simulink model "BPM_VA_Agitation_sfun_xk"  (R2022b)
settings: configuration reference "ModelConfig_var" (kept outside this file)
InitFcn:
  | %% BUS initialization
  | Xabc.A = 0;
  | Xabc.B = 0;
  | Xabc.C = 0;
  | % -------------------------------------------------------------------------
  | Simulink.Bus.createObject(Xabc)
  | XabcBus = slBus1;
  | clear slBus1
  | 
  | %% Parameter Structure initialization
  | Motor_prm_init_bpm;
model workspace (MAT data in the model file):
  Mech_HAs_CF = 0
  Mech_HAs_J_drum = 0
  Mech_HAs_TR = 0
  Mech_HAs_damp = 0
  Mech_HAs_m_unb = 0
  Mech_HAs_r_unb = 0
  Mech_VAa_J_basket = 0
  Mech_VAa_J_impeller = 0
  Mech_VAa_basket_dens = 0
  Mech_VAa_basket_dia = 0
  Mech_VAa_belt_ratio = 0
  Mech_VAa_clothes_mass = 0
  Mech_VAa_gear_ratio = 0
  Mech_VAa_imp_dens = 0
  Mech_VAa_water_vol = 0
  Mech_VAs_D_r = 0
  Mech_VAs_I_zt = 0
  Mech_VAs_K = 2700
  Mech_VAs_T_f = 0
  Mech_VAs_belt_rat = 0
  Mech_VAs_d = 0
  Mech_VAs_e = 0
  Mech_VAs_m_b1 = 0
  Mech_VAs_m_b2 = 0
  Mech_VAs_m_d = 0
  Mech_VAs_m_t = 0
  Mech_VAs_m_u = 0
  Time_step = 0.0001
  Time_step_solver = 0
  bpm_B = 0
  bpm_Ipk = [0 1 2 3 4 5 6 7]
  bpm_Jrotor = 0
  bpm_Ld_0 = 0.02117
  bpm_Ld_a = [0.02117 0.02117 0.02117 0.02117 0.02117 0.02117 0.02117 0.02117]
  bpm_Loss_Power = [0 1 2 3 4 5 6 7]
  bpm_Loss_Speed = [0 1 2 3 4 5 6 7]
  bpm_Loss_flag = 1
  bpm_Loss_th = 10
  bpm_Lq_0 = 0.02117
  bpm_Lq_b = [0.02117 0.02117 0.02117 0.02117 0.02117 0.02117 0.02117 0.02117]
  bpm_Ls_sat_flag = 1
  bpm_NPP = 0
  bpm_PM_flux_h1_0 = 0
  bpm_PM_rotor_alpha = 0
  bpm_Rs_0 = 0
  bpm_Rs_stator_alpha = 0
  bpm_Rsa_aux = 0
  bpm_Rsb_aux = 0
  bpm_Rsc_aux = 0
  bpm_TR = 1
  bpm_Temp_rotor_0 = 0
  bpm_Temp_stator_0 = 0
libraries: bpm_dq_S_noH_D_RL_U_VA_Agitation_xk x1
settings Model: ParameterArgumentNames=Mech_HAs_CF,Mech_HAs_J_drum,Mech_HAs_TR,Mech_HAs_damp,Mech_HAs_m_unb,Mech_HAs_r_unb,Mech_VAa_J_basket,Mech_VAa_J_impeller,Mech_VAa_basket_dens,Mech_VAa_basket_dia,Mech_VAa_belt_ratio,Mech_VAa_clothes_mass,Mech_VAa_gear_ratio,Mech_VAa_imp_dens,Mech_VAa_water_vol,Mech_VAs_D_r,Mech_VAs_I_zt,Mech_VAs_K,Mech_VAs_T_f,Mech_VAs_belt_rat,Mech_VAs_d,Mech_VAs_e,Mech_VAs_m_b1,Mech_VAs_m_b2,Mech_VAs_m_d,Mech_VAs_m_t,Mech_VAs_m_u,Time_step_solver,bpm_B,bpm_Ipk,bpm_Jrotor,bpm_Ld_0,bpm_Ld_a,bpm_Loss_Power,bpm_Loss_Speed,bpm_Loss_flag,bpm_Loss_th,bpm_Lq_0,bpm_Lq_b,bpm_Ls_sat_flag,bpm_NPP,bpm_PM_flux_h1_0,bpm_PM_rotor_alpha,bpm_Rs_0,bpm_Rs_stator_alpha,bpm_Rsa_aux,bpm_Rsb_aux,bpm_Rsc_aux,bpm_TR,bpm_Temp_rotor_0,bpm_Temp_stator_0  Creator=BEDNASA  LastModifiedBy=BEDNASA
settings ConfigSetRef: SourceName=ModelConfig_var  SourceLocation=Base Workspace

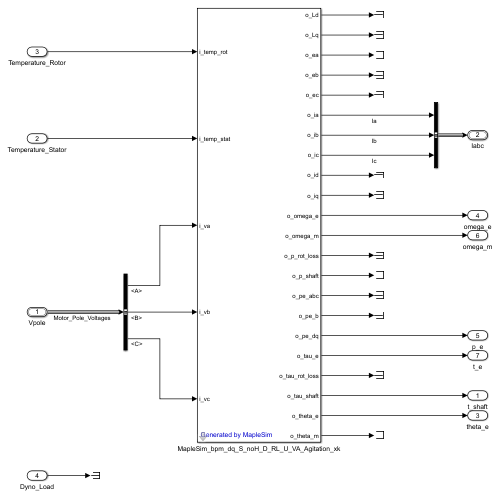
[thumbnail: Simulink's stored preview of the top-level diagram]
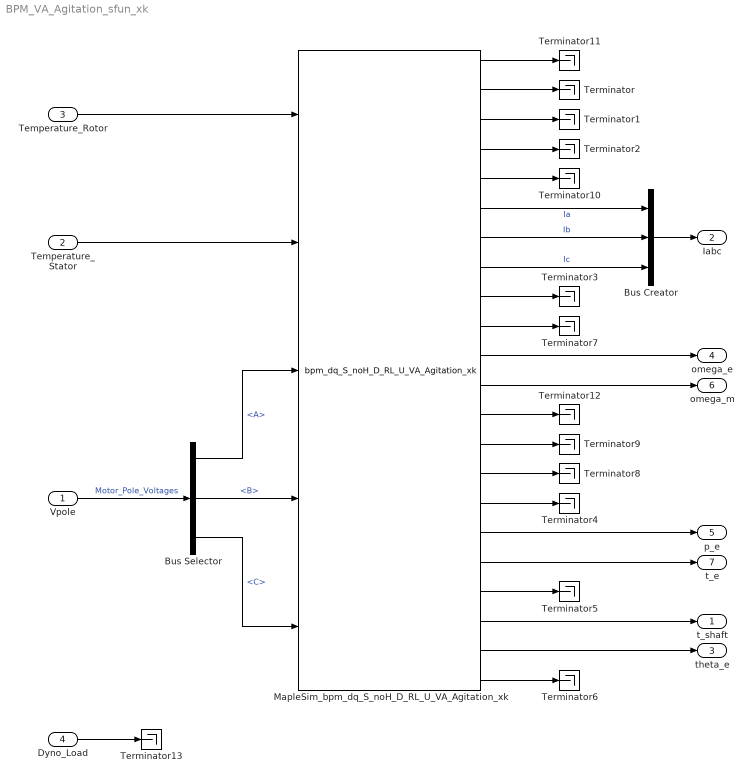
== system BPM_VA_Agitation_sfun_xk ==
  Vpole : Inport  OutDataTypeStr=Bus: XabcBus
  Temperature_Stator : Inport  Port=2
  Temperature_Rotor : Inport  Port=3
  Dyno_Load : Inport  Port=4
  Bus Creator : BusCreator  Inputs=3
  Bus Selector : BusSelector  OutputSignals=A,B,C
  MapleSim_bpm_dq_S_noH_D_RL_U_VA_Agitation_xk : bpm_dq_S_noH_D_RL_U_VA_Agitation_xk/bpm_dq_S_noH_D_RL_U_VA_Agitation_xk  Description=Subsystem: MapleSim_bpm_dq_S_noH_D_RL_U_VA_Agitation_xk  ic=[-0., 0., -0., 0., -0., 0., -0., 0., -0., 0., 0., 0., 0., 0.]  Par1=bpm_B  Par2=bpm_Ipk(1)  Par3=bpm_Ipk(2)  Par4=bpm_Ipk(3)  Par5=bpm_Ipk(4)  Par6=bpm_Ipk(5)  Par7=bpm_Ipk(6)  Par8=bpm_Ipk(7)  Par9=bpm_Ipk(8)  Par10=bpm_Jrotor  Par11=bpm_Ld_0  Par12=bpm_Ld_a(1)  Par13=bpm_Ld_a(2)  Par14=bpm_Ld_a(3)  Par15=bpm_Ld_a(4)  Par16=bpm_Ld_a(5)  Par17=bpm_Ld_a(6)  Par18=bpm_Ld_a(7)  Par19=bpm_Ld_a(8)  Par20=bpm_Lq_0  Par21=bpm_Lq_b(1)  Par22=bpm_Lq_b(2)  Par23=bpm_Lq_b(3)  Par24=bpm_Lq_b(4)  Par25=bpm_Lq_b(5)  Par26=bpm_Lq_b(6)  Par27=bpm_Lq_b(7)  Par28=bpm_Lq_b(8)  Par29=bpm_Ls_sat_flag  Par30=bpm_NPP  Par31=bpm_Loss_Power(1)  Par32=bpm_Loss_Power(2)  Par33=bpm_Loss_Power(3)  Par34=bpm_Loss_Power(4)  Par35=bpm_Loss_Power(5)  Par36=bpm_Loss_Power(6)  Par37=bpm_Loss_Power(7)  Par38=bpm_Loss_Power(8)  Par39=bpm_Loss_Speed(1)  Par40=bpm_Loss_Speed(2)  Par41=bpm_Loss_Speed(3)  Par42=bpm_Loss_Speed(4)  Par43=bpm_Loss_Speed(5)  Par44=bpm_Loss_Speed(6)  Par45=bpm_Loss_Speed(7)  Par46=bpm_Loss_Speed(8)  Par47=bpm_Loss_flag  Par48=bpm_Loss_th  Par49=bpm_Rs_0  Par50=bpm_Rsa_aux  Par51=bpm_Rsb_aux  Par52=bpm_Rsc_aux  Par53=bpm_Temp_rotor_0  Par54=bpm_Temp_stator_0  Par55=Time_step_solver  Par56=bpm_Rs_stator_alpha  Par57=bpm_PM_rotor_alpha  Par58=bpm_PM_flux_h1_0  Par59=Mech_VAa_basket_dia  Par60=Mech_VAa_clothes_mass  Par61=4.23681450081440905  Par62=5.78489261990852491  Par63=.130062059062488242  Par64=2.51144671645133697  Par65=.813472814676472229e-2  Par66=52.1060414955483938  Par67=Mech_VAa_J_basket  Par68=Mech_VAa_J_impeller  Par69=1.4270582175789073  Par70=12.0291903656936093  Par71=6.33381904348042595  Par72=2.3559208849248882  Par73=3.07609149344609313  Par74=3.16664968265920829  Par75=Mech_VAa_belt_ratio  Par76=.501051232161794397  Par77=.500198165205360073  Par78=.519008970935830595  Par79=.502279004521981584  Par80=0.  Par81=Mech_VAa_gear_ratio  Par82=0.  Par83=0.  Par84=0.  Par85=0.  Par86=0.  Par87=0.  Par88=Mech_VAa_water_vol  MinStep=1/40  TimeStep_Solver=TimeSteps.ModelStep
      settings: LibrarySourceBlock=MapleSim_bpm_dq_S_noH_D_RL_U_VA_Agitation_xk/MapleSim_bpm_dq_S_noH_D_RL_U_VA_Agitation_xk
  Terminator{,1..13} (14 alike) : Terminator
  t_shaft : Outport  VectorParamsAs1DForOutWhenUnconnected=off
  Iabc : Outport  Port=2  OutDataTypeStr=Bus: XabcBus  VectorParamsAs1DForOutWhenUnconnected=off
  theta_e : Outport  Port=3  VectorParamsAs1DForOutWhenUnconnected=off
  omega_e : Outport  Port=4  VectorParamsAs1DForOutWhenUnconnected=off
  p_e : Outport  Port=5  VectorParamsAs1DForOutWhenUnconnected=off
  omega_m : Outport  Port=6  VectorParamsAs1DForOutWhenUnconnected=off
  t_e : Outport  Port=7  VectorParamsAs1DForOutWhenUnconnected=off
  wires:
  MapleSim_bpm_dq_S_noH_D_RL_U_VA_Agitation_xk/2 -> Terminator/1
  MapleSim_bpm_dq_S_noH_D_RL_U_VA_Agitation_xk/3 -> Terminator1/1
  MapleSim_bpm_dq_S_noH_D_RL_U_VA_Agitation_xk/4 -> Terminator2/1
  MapleSim_bpm_dq_S_noH_D_RL_U_VA_Agitation_xk/9 -> Terminator3/1
  MapleSim_bpm_dq_S_noH_D_RL_U_VA_Agitation_xk/16 -> Terminator4/1
  MapleSim_bpm_dq_S_noH_D_RL_U_VA_Agitation_xk/12 -> omega_m/1
  MapleSim_bpm_dq_S_noH_D_RL_U_VA_Agitation_xk/11 -> omega_e/1
  MapleSim_bpm_dq_S_noH_D_RL_U_VA_Agitation_xk/21 -> theta_e/1
  MapleSim_bpm_dq_S_noH_D_RL_U_VA_Agitation_xk/18 -> t_e/1
  MapleSim_bpm_dq_S_noH_D_RL_U_VA_Agitation_xk/20 -> t_shaft/1
  MapleSim_bpm_dq_S_noH_D_RL_U_VA_Agitation_xk/19 -> Terminator5/1
  MapleSim_bpm_dq_S_noH_D_RL_U_VA_Agitation_xk/22 -> Terminator6/1
  MapleSim_bpm_dq_S_noH_D_RL_U_VA_Agitation_xk/10 -> Terminator7/1
  MapleSim_bpm_dq_S_noH_D_RL_U_VA_Agitation_xk/17 -> p_e/1
  MapleSim_bpm_dq_S_noH_D_RL_U_VA_Agitation_xk/15 -> Terminator8/1
  MapleSim_bpm_dq_S_noH_D_RL_U_VA_Agitation_xk/5 -> Terminator10/1
  MapleSim_bpm_dq_S_noH_D_RL_U_VA_Agitation_xk/1 -> Terminator11/1
  Bus Selector/3 -> MapleSim_bpm_dq_S_noH_D_RL_U_VA_Agitation_xk/5  "<C>"
  Bus Selector/2 -> MapleSim_bpm_dq_S_noH_D_RL_U_VA_Agitation_xk/4  "<B>"
  Vpole/1 -> Bus Selector/1  "Motor_Pole_Voltages"
  MapleSim_bpm_dq_S_noH_D_RL_U_VA_Agitation_xk/7 -> Bus Creator/2  "Ib"
  Bus Creator/1 -> Iabc/1
  MapleSim_bpm_dq_S_noH_D_RL_U_VA_Agitation_xk/6 -> Bus Creator/1  "Ia"
  MapleSim_bpm_dq_S_noH_D_RL_U_VA_Agitation_xk/8 -> Bus Creator/3  "Ic"
  Bus Selector/1 -> MapleSim_bpm_dq_S_noH_D_RL_U_VA_Agitation_xk/3  "<A>"
  MapleSim_bpm_dq_S_noH_D_RL_U_VA_Agitation_xk/13 -> Terminator12/1
  MapleSim_bpm_dq_S_noH_D_RL_U_VA_Agitation_xk/14 -> Terminator9/1
  Temperature_Stator/1 -> MapleSim_bpm_dq_S_noH_D_RL_U_VA_Agitation_xk/2
  Temperature_Rotor/1 -> MapleSim_bpm_dq_S_noH_D_RL_U_VA_Agitation_xk/1
  Dyno_Load/1 -> Terminator13/1
